simulink model "Complete_Model_Tests"  (R2023b)
settings: Solver=VariableStepAuto  StartTime=0.0  StopTime=10  RelTol=1e-3
values from neighbouring files (symbols this model uses):
  b = 1.5    [Parameters.m]
  Csc = 600    [Parameters.m]
  Cse = 1200    [Parameters.m]
  g = 9.81    [Parameters.m]
  I = 650    [Parameters.m]
  Ks = 2e4    (= 20000)    [Parameters.m]
  Kt = 14e4    (= 140000)    [Parameters.m]
  Mw = 20    [Parameters.m]
libraries: CarModelLibrary x26, simulink x4
settings Model: Creator=fb552  LastModifiedBy=franc
settings SolverCC: AlgebraicLoopSolver=TrustRegion
settings DebuggingCC: UnconnectedInputMsg=warning  UnconnectedOutputMsg=warning  UnconnectedLineMsg=warning
settings ModelReferenceCC: EnableRefExpFcnMdlSchedulingChecks=on

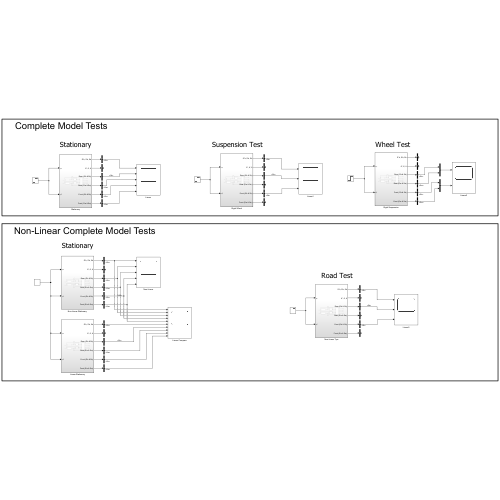
[thumbnail: Simulink's stored preview of the top-level diagram]
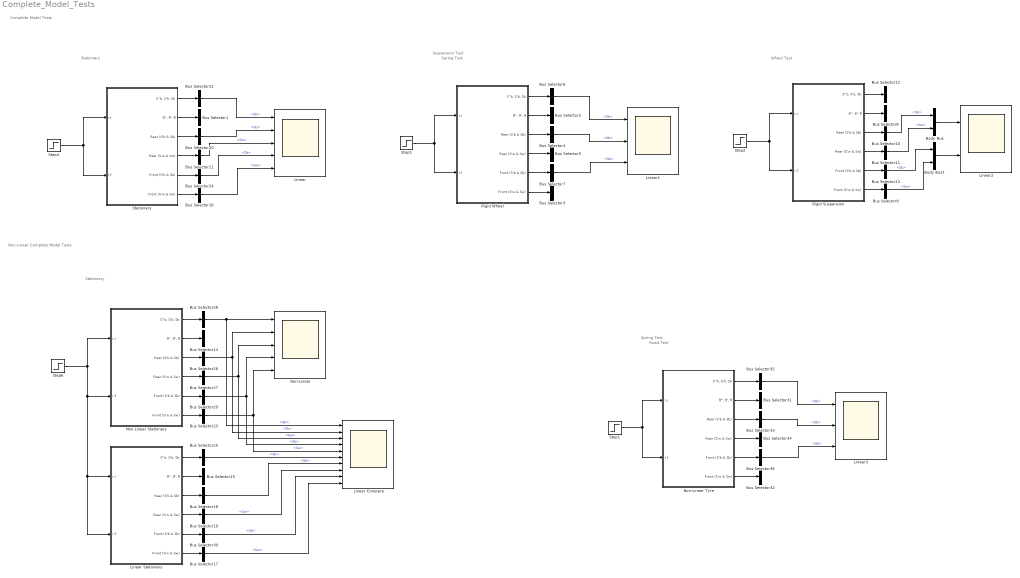
== system Complete_Model_Tests ==
  note: Complete Model Tests
  note: Stationary
  note: Spring Test
  note: Wheel Test
  note: Suspension Test
  note: Stationary
  note: Non-Linear Complete Model Tests
  note: Road Test
  note: Spring Test
  Body Bus : BusCreator  Inputs=2
  Body Bus1 : BusCreator  Inputs=2
  Bus Selector{1..2,8,14..15,31} (6 alike) : BusSelector  OutputSignals=θ
  Bus Selector{4,6..7,10,12..13,18,20,22,24..26,28..30,33,35..36} (18 alike) : BusSelector  OutputSignals=Sb
  Bus Selector{3,5,9,11,16..17,19,21,23,27,32,34} (12 alike) : BusSelector  OutputSignals=Sw
  Linear : Scope  NumInputPorts=5
  Linear Compare : Scope  NumInputPorts=10
  Linear Stationary : Subsystem
  Linear1 : Scope  NumInputPorts=3
  Linear2 : Scope  NumInputPorts=2
  Linear3 : Scope  NumInputPorts=3
  Non-Linear : Scope  NumInputPorts=5
  "Non-Linear Stationary " : Subsystem
  Non-Linear Tyre : Subsystem
  Rigid Suspension : Subsystem
  Rigid Wheel : Subsystem
  Stationary : Subsystem
  Step1 : Step  SampleTime=0
  Step2 : Step  SampleTime=0
  Step3 : Step  SampleTime=0
  Step4 : Step  Time=0  After=0  SampleTime=0
  Step6 : Step  Time=0  After=0  SampleTime=0
  wires:
  Bus Selector22/1 -> Linear/1  "<Sb>"
  Stationary/1("S''b, S'b, Sb") -> Bus Selector22/1
  Stationary/6(Front (S'w & Sw)) -> Bus Selector16/1
  Stationary/5(Front (S'b & Sb)) -> Bus Selector24/1
  Stationary/4(Rear (S'w & Sw)) -> Bus Selector21/1
  Step4/1 -> Stationary/1(r,r), Stationary/2(r,f)
  Stationary/3(Rear (S'b & Sb)) -> Bus Selector20/1
  Bus Selector24/1 -> Linear/4  "<Sb>"
  Bus Selector20/1 -> Linear/2  "<Sb>"
  Stationary/2("θ'', θ', θ") -> Bus Selector1/1
  Bus Selector16/1 -> Linear/5  "<Sw>"
  Bus Selector21/1 -> Linear/3  "<Sw>"
  Rigid Wheel/3(Rear (S'b & Sb)) -> Bus Selector4/1
  Bus Selector7/1 -> Linear1/3  "<Sb>"
  Bus Selector4/1 -> Linear1/2  "<Sb>"
  Bus Selector6/1 -> Linear1/1  "<Sb>"
  Rigid Wheel/2("θ'', θ', θ") -> Bus Selector2/1
  Step3/1 -> Rigid Wheel/1(r,r), Rigid Wheel/2(r,f)
  Rigid Wheel/4(Rear (S'w & Sw)) -> Bus Selector5/1
  Rigid Wheel/1("S''b, S'b, Sb") -> Bus Selector6/1
  Rigid Wheel/6(Front (S'w & Sw)) -> Bus Selector3/1
  Rigid Wheel/5(Front (S'b & Sb)) -> Bus Selector7/1
  Rigid Suspension/6(Front (S'w & Sw)) -> Bus Selector9/1
  Rigid Suspension/5(Front (S'b & Sb)) -> Bus Selector13/1
  Rigid Suspension/1("S''b, S'b, Sb") -> Bus Selector12/1
  Step2/1 -> Rigid Suspension/1(r,r), Rigid Suspension/2(r,f)
  Rigid Suspension/2("θ'', θ', θ") -> Bus Selector8/1
  Rigid Suspension/3(Rear (S'b & Sb)) -> Bus Selector10/1
  Rigid Suspension/4(Rear (S'w & Sw)) -> Bus Selector11/1
  Bus Selector10/1 -> Body Bus/1  "<Sb>"
  Bus Selector11/1 -> Body Bus/2  "<Sw>"
  Body Bus/1 -> Linear2/1
  Body Bus1/1 -> Linear2/2
  Bus Selector9/1 -> Body Bus1/2  "<Sw>"
  Bus Selector13/1 -> Body Bus1/1  "<Sb>"
  "Non-Linear Stationary "/2("θ'', θ', θ") -> Bus Selector14/1
  "Non-Linear Stationary "/4(Rear (S'w & Sw)) -> Bus Selector27/1
  Bus Selector26/1 -> Non-Linear/2, Linear Compare/2  "<Sb>"
  Bus Selector23/1 -> Non-Linear/5, Linear Compare/5  "<Sw>"
  "Non-Linear Stationary "/6(Front (S'w & Sw)) -> Bus Selector23/1
  Bus Selector29/1 -> Non-Linear/4, Linear Compare/4  "<Sb>"
  Bus Selector27/1 -> Non-Linear/3, Linear Compare/3  "<Sw>"
  "Non-Linear Stationary "/3(Rear (S'b & Sb)) -> Bus Selector26/1
  "Non-Linear Stationary "/1("S''b, S'b, Sb") -> Bus Selector28/1
  Bus Selector28/1 -> Non-Linear/1, Linear Compare/1  "<Sb>"
  "Non-Linear Stationary "/5(Front (S'b & Sb)) -> Bus Selector29/1
  Linear Stationary/2("θ'', θ', θ") -> Bus Selector15/1
  Linear Stationary/4(Rear (S'w & Sw)) -> Bus Selector19/1
  Bus Selector18/1 -> Linear Compare/7  "<Sb>"
  Bus Selector17/1 -> Linear Compare/10  "<Sw>"
  Linear Stationary/6(Front (S'w & Sw)) -> Bus Selector17/1
  Bus Selector30/1 -> Linear Compare/9  "<Sb>"
  Linear Stationary/1("S''b, S'b, Sb") -> Bus Selector25/1
  Linear Stationary/3(Rear (S'b & Sb)) -> Bus Selector18/1
  Bus Selector19/1 -> Linear Compare/8  "<Sw>"
  Bus Selector25/1 -> Linear Compare/6  "<Sb>"
  Linear Stationary/5(Front (S'b & Sb)) -> Bus Selector30/1
  Step6/1 -> "Non-Linear Stationary "/1(r,r), Linear Stationary/1(r,r), Linear Stationary/2(r,f), "Non-Linear Stationary "/2(r,f)
  Non-Linear Tyre/3(Rear (S'b & Sb)) -> Bus Selector33/1
  Non-Linear Tyre/5(Front (S'b & Sb)) -> Bus Selector36/1
  Non-Linear Tyre/1("S''b, S'b, Sb") -> Bus Selector35/1
  Non-Linear Tyre/4(Rear (S'w & Sw)) -> Bus Selector34/1
  Non-Linear Tyre/2("θ'', θ', θ") -> Bus Selector31/1
  Bus Selector36/1 -> Linear3/3  "<Sb>"
  Bus Selector33/1 -> Linear3/2  "<Sb>"
  Non-Linear Tyre/6(Front (S'w & Sw)) -> Bus Selector32/1
  Bus Selector35/1 -> Linear3/1  "<Sb>"
  Step1/1 -> Non-Linear Tyre/2(r,f), Non-Linear Tyre/1(r,r)

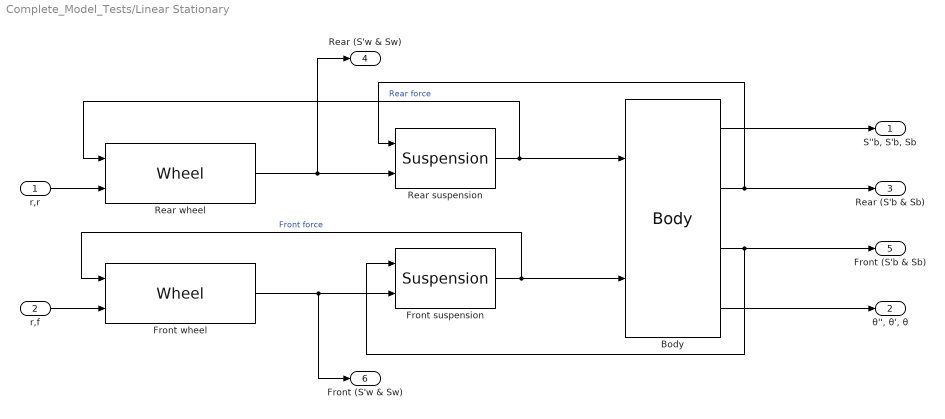
== system Complete_Model_Tests/Linear Stationary ==
  r,r : Inport
  r,f : Inport  Port=2
  Body : CarModelLibrary/Body  mb=Mb  I=I  a=a  b=b
  Front suspension : CarModelLibrary/Suspension  ks=Ks  ksstiff=1  x0=x0  csb=(Csc+Cse)/2  csr=(Csc+Cse)/2
  Front wheel : CarModelLibrary/Wheel  mw=Mw  Kt=Kt  g=g
  Rear suspension : CarModelLibrary/Suspension  ks=Ks  ksstiff=1  x0=x0  csb=(Csc+Cse)/2  csr=(Csc+Cse)/2
  Rear wheel : CarModelLibrary/Wheel  mw=Mw  Kt=Kt  g=g
  "S''b, S'b, Sb" : Outport
  "θ'', θ', θ" : Outport  Port=2
  Rear (S'b & Sb) : Outport  Port=3
  Rear (S'w & Sw) : Outport  Port=4
  Front (S'b & Sb) : Outport  Port=5
  Front (S'w & Sw) : Outport  Port=6
  wires:
  Body/1 -> "S''b, S'b, Sb"/1
  Body/2 -> Rear suspension/1, Rear (S'b & Sb)/1
  Front wheel/1 -> Front suspension/2, Front (S'w & Sw)/1
  Rear wheel/1 -> Rear suspension/2, Rear (S'w & Sw)/1
  Body/4 -> "θ'', θ', θ"/1
  Body/3 -> Front suspension/1, Front (S'b & Sb)/1
  Rear suspension/1 -> Body/1, Rear wheel/1  "Rear force"
  r,r/1 -> Rear wheel/2
  r,f/1 -> Front wheel/2
  Front suspension/1 -> Front wheel/1, Body/2  "Front force"

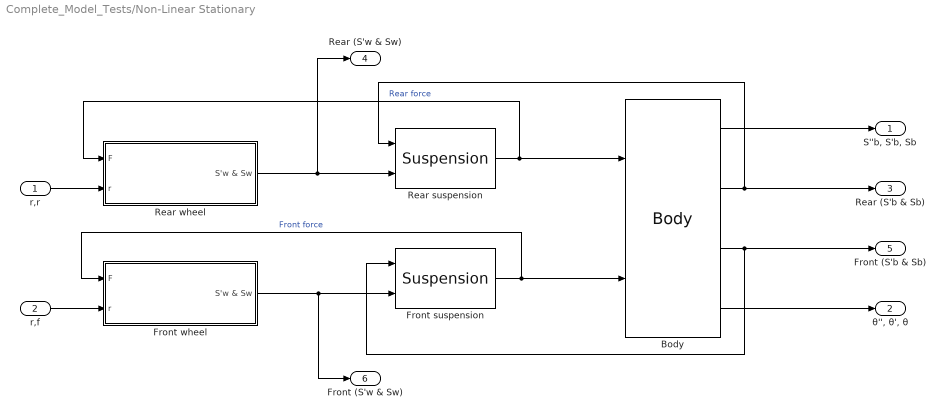
== system Complete_Model_Tests/Non-Linear Stationary  ==
  r,r : Inport
  r,f : Inport  Port=2
  Body : CarModelLibrary/Body  mb=Mb  I=I  a=a  b=b
  Front suspension : CarModelLibrary/Suspension  ks=Ks  ksstiff=Kstiff  x0=x0  csb=Csc  csr=Cse
  Front wheel : Subsystem  AncestorBlock=CarModelLibrary/Wheel  mask{mw=Mw, Kt=Kt, g=9.81}
      mask prompts: mw "Wheel Mass (Kg)"; Kt "Tyre Stiffness"; g "Gravitational acceleration"
  Rear suspension : CarModelLibrary/Suspension  ks=Ks  ksstiff=Kstiff  x0=x0  csb=Csc  csr=Cse
  Rear wheel : Subsystem  AncestorBlock=CarModelLibrary/Wheel  mask{mw=Mw, Kt=Kt, g=9.81}
      mask prompts: mw "Wheel Mass (Kg)"; Kt "Tyre Stiffness"; g "Gravitational acceleration"
  "S''b, S'b, Sb" : Outport
  "θ'', θ', θ" : Outport  Port=2
  Rear (S'b & Sb) : Outport  Port=3
  Rear (S'w & Sw) : Outport  Port=4
  Front (S'b & Sb) : Outport  Port=5
  Front (S'w & Sw) : Outport  Port=6
  wires:
  Body/1 -> "S''b, S'b, Sb"/1
  Body/2 -> Rear suspension/1, Rear (S'b & Sb)/1
  Front wheel/1(S'w & Sw) -> Front suspension/2, Front (S'w & Sw)/1
  Rear wheel/1(S'w & Sw) -> Rear suspension/2, Rear (S'w & Sw)/1
  Body/4 -> "θ'', θ', θ"/1
  Body/3 -> Front suspension/1, Front (S'b & Sb)/1
  Rear suspension/1 -> Body/1, Rear wheel/1(F)  "Rear force"
  r,r/1 -> Rear wheel/2(r)
  r,f/1 -> Front wheel/2(r)
  Front suspension/1 -> Front wheel/1(F), Body/2  "Front force"

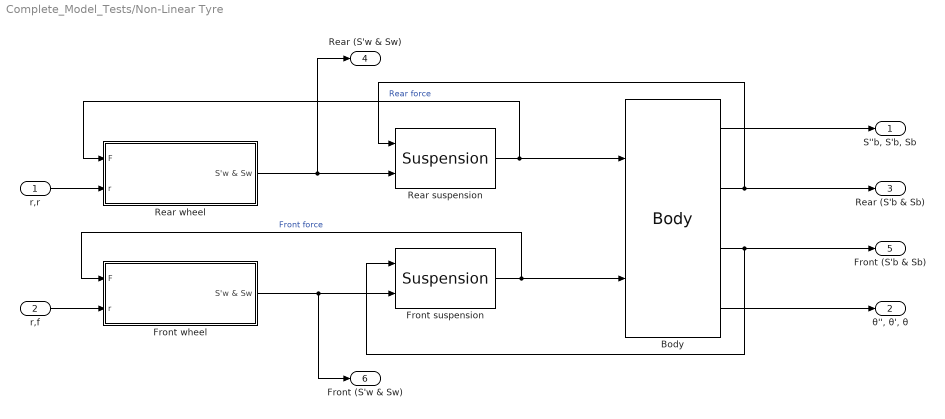
== system Complete_Model_Tests/Non-Linear Tyre ==
  r,r : Inport
  r,f : Inport  Port=2
  Body : CarModelLibrary/Body  mb=Mb  I=I  a=a  b=b
  Front suspension : CarModelLibrary/Suspension  ks=Ks  ksstiff=Kstiff  x0=x0  csb=Cse  csr=Csc
  Front wheel : Subsystem  AncestorBlock=CarModelLibrary/Wheel  mask{mw=Mw, Kt=Kt, g=9.81}
      mask prompts: mw "Wheel Mass (Kg)"; Kt "Tyre Stiffness"; g "Gravitational acceleration"
  Rear suspension : CarModelLibrary/Suspension  ks=Ks  ksstiff=Kstiff  x0=x0  csb=Csc  csr=Cse
  Rear wheel : Subsystem  AncestorBlock=CarModelLibrary/Wheel  mask{mw=Mw, Kt=Kt, g=9.81}
      mask prompts: mw "Wheel Mass (Kg)"; Kt "Tyre Stiffness"; g "Gravitational acceleration"
  "S''b, S'b, Sb" : Outport
  "θ'', θ', θ" : Outport  Port=2
  Rear (S'b & Sb) : Outport  Port=3
  Rear (S'w & Sw) : Outport  Port=4
  Front (S'b & Sb) : Outport  Port=5
  Front (S'w & Sw) : Outport  Port=6
  wires:
  Body/1 -> "S''b, S'b, Sb"/1
  Body/2 -> Rear suspension/1, Rear (S'b & Sb)/1
  Front wheel/1(S'w & Sw) -> Front suspension/2, Front (S'w & Sw)/1
  Rear wheel/1(S'w & Sw) -> Rear suspension/2, Rear (S'w & Sw)/1
  Body/4 -> "θ'', θ', θ"/1
  Body/3 -> Front suspension/1, Front (S'b & Sb)/1
  Rear suspension/1 -> Body/1, Rear wheel/1(F)  "Rear force"
  r,r/1 -> Rear wheel/2(r)
  r,f/1 -> Front wheel/2(r)
  Front suspension/1 -> Front wheel/1(F), Body/2  "Front force"

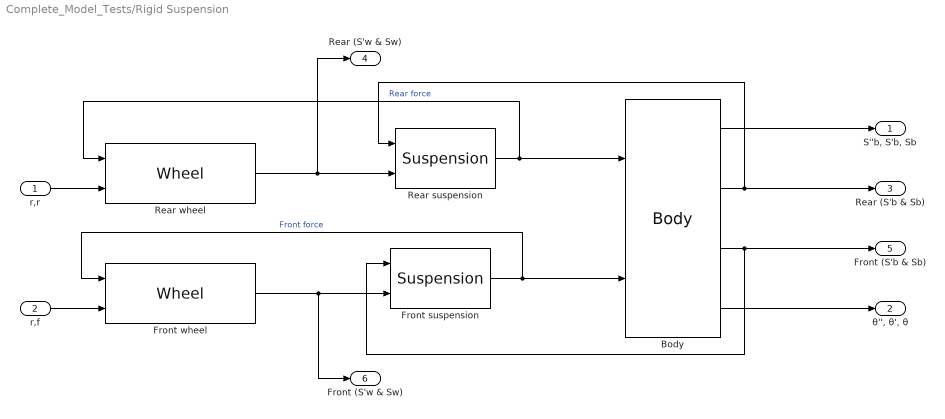
== system Complete_Model_Tests/Rigid Suspension ==
  r,r : Inport
  r,f : Inport  Port=2
  Body : CarModelLibrary/Body  mb=Mb  I=I  a=a  b=b
  Front suspension : CarModelLibrary/Suspension  ks=Ks*1e6  ksstiff=1  x0=x0  csb=(Csc+Cse)/2*1e8  csr=(Csc+Cse)/2*1e8
  Front wheel : CarModelLibrary/Wheel  mw=Mw  Kt=Kt  g=g
  Rear suspension : CarModelLibrary/Suspension  ks=Ks*1e6  ksstiff=1  x0=x0  csb=(Csc+Cse)/2*1e8  csr=(Csc+Cse)/2*1e8
  Rear wheel : CarModelLibrary/Wheel  mw=Mw  Kt=Kt  g=g
  "S''b, S'b, Sb" : Outport
  "θ'', θ', θ" : Outport  Port=2
  Rear (S'b & Sb) : Outport  Port=3
  Rear (S'w & Sw) : Outport  Port=4
  Front (S'b & Sb) : Outport  Port=5
  Front (S'w & Sw) : Outport  Port=6
  wires:
  Body/1 -> "S''b, S'b, Sb"/1
  Body/2 -> Rear suspension/1, Rear (S'b & Sb)/1
  Front wheel/1 -> Front suspension/2, Front (S'w & Sw)/1
  Rear wheel/1 -> Rear suspension/2, Rear (S'w & Sw)/1
  Body/4 -> "θ'', θ', θ"/1
  Body/3 -> Front suspension/1, Front (S'b & Sb)/1
  Rear suspension/1 -> Body/1, Rear wheel/1  "Rear force"
  r,r/1 -> Rear wheel/2
  r,f/1 -> Front wheel/2
  Front suspension/1 -> Front wheel/1, Body/2  "Front force"

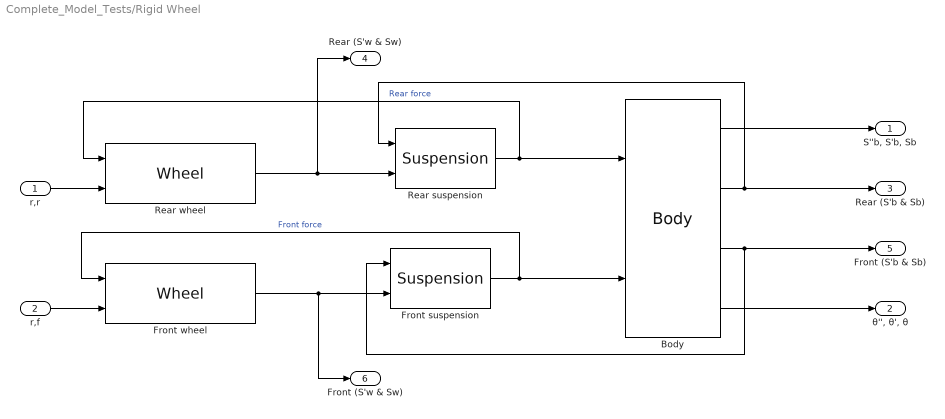
== system Complete_Model_Tests/Rigid Wheel ==
  r,r : Inport
  r,f : Inport  Port=2
  Body : CarModelLibrary/Body  mb=Mb  I=I  a=a  b=b
  Front suspension : CarModelLibrary/Suspension  ks=Ks  ksstiff=1  x0=x0  csb=(Csc+Cse)/2  csr=(Csc+Cse)/2
  Front wheel : CarModelLibrary/Wheel  mw=Mw/10000  Kt=Kt*10000  g=g
  Rear suspension : CarModelLibrary/Suspension  ks=Ks  ksstiff=1  x0=x0  csb=(Csc+Cse)/2  csr=(Csc+Cse)/2
  Rear wheel : CarModelLibrary/Wheel  mw=Mw/10000  Kt=Kt*10000  g=g
  "S''b, S'b, Sb" : Outport
  "θ'', θ', θ" : Outport  Port=2
  Rear (S'b & Sb) : Outport  Port=3
  Rear (S'w & Sw) : Outport  Port=4
  Front (S'b & Sb) : Outport  Port=5
  Front (S'w & Sw) : Outport  Port=6
  wires:
  Body/1 -> "S''b, S'b, Sb"/1
  Body/2 -> Rear suspension/1, Rear (S'b & Sb)/1
  Front wheel/1 -> Front suspension/2, Front (S'w & Sw)/1
  Rear wheel/1 -> Rear suspension/2, Rear (S'w & Sw)/1
  Body/4 -> "θ'', θ', θ"/1
  Body/3 -> Front suspension/1, Front (S'b & Sb)/1
  Rear suspension/1 -> Body/1, Rear wheel/1  "Rear force"
  r,r/1 -> Rear wheel/2
  r,f/1 -> Front wheel/2
  Front suspension/1 -> Front wheel/1, Body/2  "Front force"

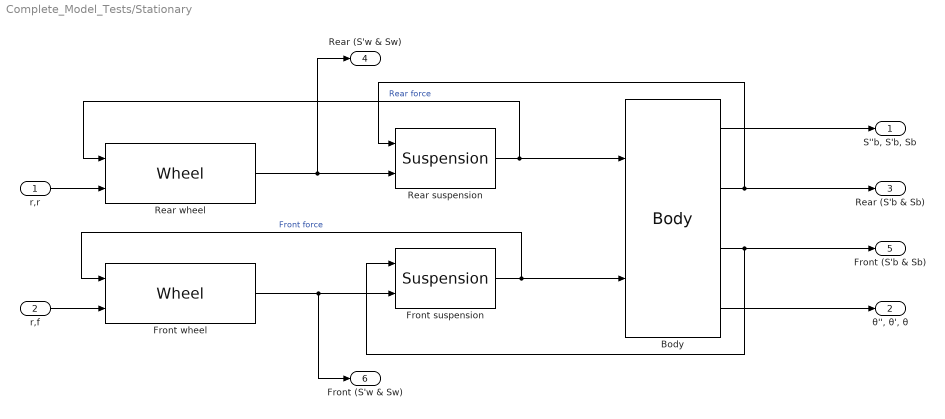
== system Complete_Model_Tests/Stationary ==
  r,r : Inport
  r,f : Inport  Port=2
  Body : CarModelLibrary/Body  mb=Mb  I=I  a=a  b=b
  Front suspension : CarModelLibrary/Suspension  ks=Ks  ksstiff=1  x0=x0  csb=(Csc+Cse)/2  csr=(Csc+Cse)/2
  Front wheel : CarModelLibrary/Wheel  mw=Mw  Kt=Kt  g=g
  Rear suspension : CarModelLibrary/Suspension  ks=Ks  ksstiff=1  x0=x0  csb=(Csc+Cse)/2  csr=(Csc+Cse)/2
  Rear wheel : CarModelLibrary/Wheel  mw=Mw  Kt=Kt  g=g
  "S''b, S'b, Sb" : Outport
  "θ'', θ', θ" : Outport  Port=2
  Rear (S'b & Sb) : Outport  Port=3
  Rear (S'w & Sw) : Outport  Port=4
  Front (S'b & Sb) : Outport  Port=5
  Front (S'w & Sw) : Outport  Port=6
  wires:
  Body/1 -> "S''b, S'b, Sb"/1
  Body/2 -> Rear suspension/1, Rear (S'b & Sb)/1
  Front wheel/1 -> Front suspension/2, Front (S'w & Sw)/1
  Rear wheel/1 -> Rear suspension/2, Rear (S'w & Sw)/1
  Body/4 -> "θ'', θ', θ"/1
  Body/3 -> Front suspension/1, Front (S'b & Sb)/1
  Rear suspension/1 -> Body/1, Rear wheel/1  "Rear force"
  r,r/1 -> Rear wheel/2
  r,f/1 -> Front wheel/2
  Front suspension/1 -> Front wheel/1, Body/2  "Front force"

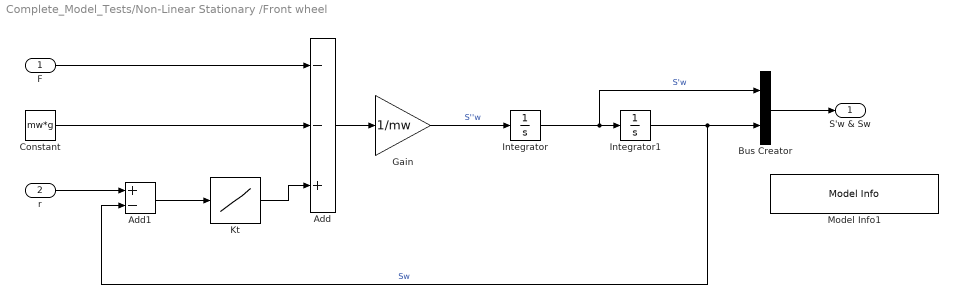
== system Complete_Model_Tests/Non-Linear Stationary /Front wheel ==
  F : Inport
  r : Inport  Port=2
  Add : Sum  Inputs=--+
  Add1 : Sum  Inputs=+-
  Bus Creator : BusCreator  Inputs=2
  Constant : Constant  Value=mw*g
  Gain : Gain  Gain=1/mw
  Integrator : Integrator
  Integrator1 : Integrator
  Kt : Lookup_n-D  NumberOfTableDimensions=1  BreakpointsForDimension1=[-1, 0, 1]  Table=[0, 0, Kt]  InternalRulePriority=Speed  RndMeth=Simplest
  Model Info1 : simulink/Model-Wide Utilities/Model Info  Frame=on  DisplayStringWithTags=m * S''w = -F + Kt (r-S) - m*g  HorizontalTextAlignment=Center  LeftAlignmentValue=0.5
  S'w & Sw : Outport
  wires:
  Kt/1 -> Add/3
  F/1 -> Add/1
  Constant/1 -> Add/2
  Gain/1 -> Integrator/1  "S''w"
  Add/1 -> Gain/1
  Integrator1/1 -> Add1/2, Bus Creator/2  "Sw"
  Bus Creator/1 -> S'w & Sw/1
  Integrator/1 -> Integrator1/1, Bus Creator/1  "S'w"
  Add1/1 -> Kt/1
  r/1 -> Add1/1

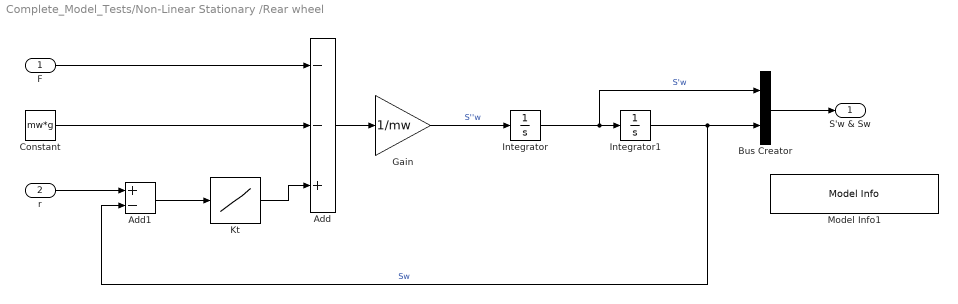
== system Complete_Model_Tests/Non-Linear Stationary /Rear wheel ==
  F : Inport
  r : Inport  Port=2
  Add : Sum  Inputs=--+
  Add1 : Sum  Inputs=+-
  Bus Creator : BusCreator  Inputs=2
  Constant : Constant  Value=mw*g
  Gain : Gain  Gain=1/mw
  Integrator : Integrator
  Integrator1 : Integrator
  Kt : Lookup_n-D  NumberOfTableDimensions=1  BreakpointsForDimension1=[-1, 0, 1]  Table=[0, 0, Kt]  InternalRulePriority=Speed  RndMeth=Simplest
  Model Info1 : simulink/Model-Wide Utilities/Model Info  Frame=on  DisplayStringWithTags=m * S''w = -F + Kt (r-S) - m*g  HorizontalTextAlignment=Center  LeftAlignmentValue=0.5
  S'w & Sw : Outport
  wires:
  Kt/1 -> Add/3
  F/1 -> Add/1
  Constant/1 -> Add/2
  Gain/1 -> Integrator/1  "S''w"
  Add/1 -> Gain/1
  Integrator1/1 -> Add1/2, Bus Creator/2  "Sw"
  Bus Creator/1 -> S'w & Sw/1
  Integrator/1 -> Integrator1/1, Bus Creator/1  "S'w"
  Add1/1 -> Kt/1
  r/1 -> Add1/1

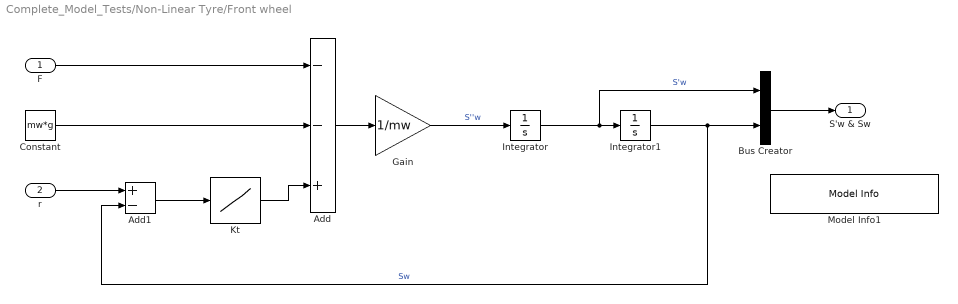
== system Complete_Model_Tests/Non-Linear Tyre/Front wheel ==
  F : Inport
  r : Inport  Port=2
  Add : Sum  Inputs=--+
  Add1 : Sum  Inputs=+-
  Bus Creator : BusCreator  Inputs=2
  Constant : Constant  Value=mw*g
  Gain : Gain  Gain=1/mw
  Integrator : Integrator
  Integrator1 : Integrator
  Kt : Lookup_n-D  NumberOfTableDimensions=1  BreakpointsForDimension1=[-1, 0, 1]  Table=[0, 0, Kt]  InternalRulePriority=Speed  RndMeth=Simplest
  Model Info1 : simulink/Model-Wide Utilities/Model Info  Frame=on  DisplayStringWithTags=m * S''w = -F + Kt (r-S) - m*g  HorizontalTextAlignment=Center  LeftAlignmentValue=0.5
  S'w & Sw : Outport
  wires:
  Kt/1 -> Add/3
  F/1 -> Add/1
  Constant/1 -> Add/2
  Gain/1 -> Integrator/1  "S''w"
  Add/1 -> Gain/1
  Integrator1/1 -> Add1/2, Bus Creator/2  "Sw"
  Bus Creator/1 -> S'w & Sw/1
  Integrator/1 -> Integrator1/1, Bus Creator/1  "S'w"
  Add1/1 -> Kt/1
  r/1 -> Add1/1

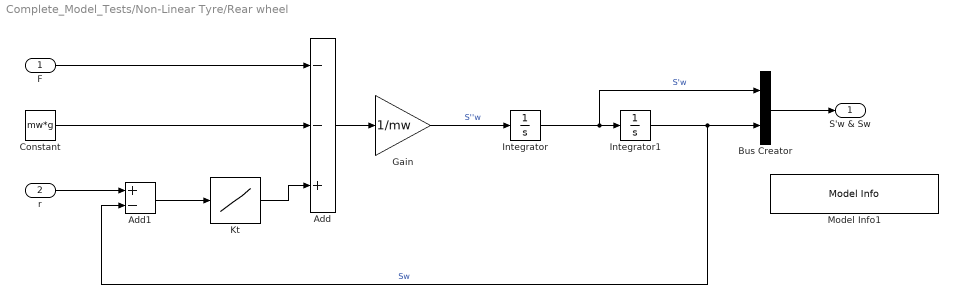
== system Complete_Model_Tests/Non-Linear Tyre/Rear wheel ==
  F : Inport
  r : Inport  Port=2
  Add : Sum  Inputs=--+
  Add1 : Sum  Inputs=+-
  Bus Creator : BusCreator  Inputs=2
  Constant : Constant  Value=mw*g
  Gain : Gain  Gain=1/mw
  Integrator : Integrator
  Integrator1 : Integrator
  Kt : Lookup_n-D  NumberOfTableDimensions=1  BreakpointsForDimension1=[-1, 0, 1]  Table=[0, 0, Kt]  InternalRulePriority=Speed  RndMeth=Simplest
  Model Info1 : simulink/Model-Wide Utilities/Model Info  Frame=on  DisplayStringWithTags=m * S''w = -F + Kt (r-S) - m*g  HorizontalTextAlignment=Center  LeftAlignmentValue=0.5
  S'w & Sw : Outport
  wires:
  Kt/1 -> Add/3
  F/1 -> Add/1
  Constant/1 -> Add/2
  Gain/1 -> Integrator/1  "S''w"
  Add/1 -> Gain/1
  Integrator1/1 -> Add1/2, Bus Creator/2  "Sw"
  Bus Creator/1 -> S'w & Sw/1
  Integrator/1 -> Integrator1/1, Bus Creator/1  "S'w"
  Add1/1 -> Kt/1
  r/1 -> Add1/1
